simulink model "SimulacionPenduloSimpleFuzzyController"  (R2024b)
settings: Solver=ode45  StartTime=0.0  StopTime=20  RelTol=1e-3
libraries: fuzblock x1
settings Model: Creator=Lenovo  LastModifiedBy=Lenovo

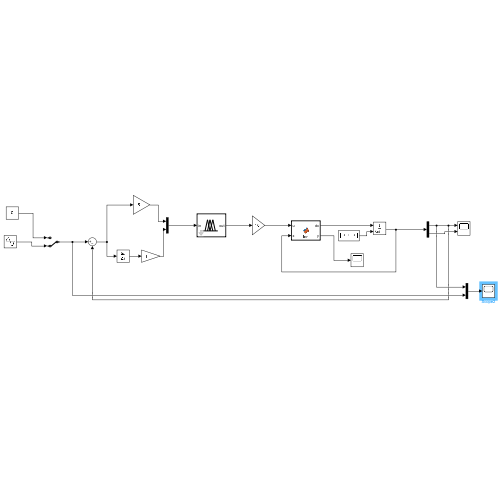
[thumbnail: Simulink's stored preview of the top-level diagram]
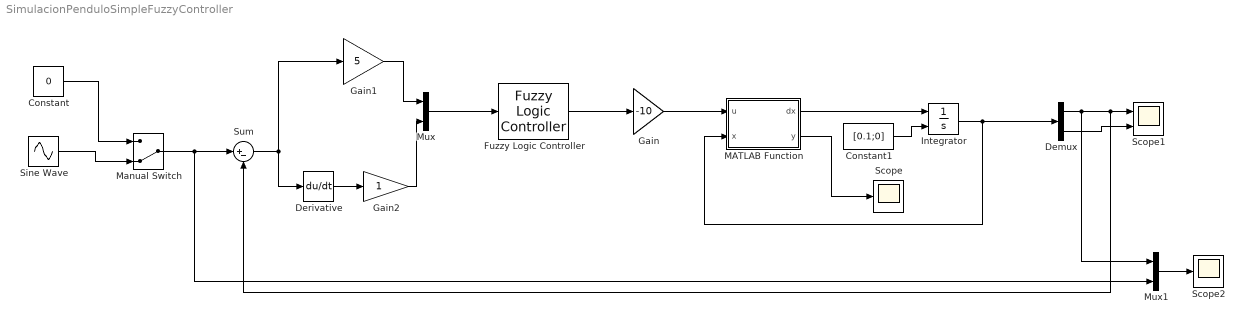
== system SimulacionPenduloSimpleFuzzyController ==
  Constant : Constant  Value=0
  Constant1 : Constant  Value=[0.1;0]
  Demux : Demux  Outputs=2
  Derivative : Derivative
  Fuzzy Logic Controller : fuzblock/Fuzzy Logic  Controller  FIS='D:\02. UP\Especialidad 1\Control difuso\Semana 05\Fuzzy5x5.fis'  OutputSampleNumber=101  DataType=double  FuzzifiedInputs=off  RuleFiringStrengths=off  RuleOutputs=off  AggregatedOutputs=off  SimulateUsing=Interpreted execution  OutOfRangeInputValueMessage=warning  NoRuleFiredMessage=warning  EmptyOutputFuzzySetMessage=warning
  Gain : Gain  Gain=-10
  Gain1 : Gain  Gain=5
  Gain2 : Gain
  Integrator : Integrator  InitialConditionSource=external
  MATLAB Function : MATLAB Function  TreatAsAtomicUnit=on
  Manual Switch : ManualSwitch  CurrentSetting=0
  Mux : Mux  Inputs=2
  Mux1 : Mux  Inputs=2
  Scope : Scope
  Scope1 : Scope  NumInputPorts=2
  Scope2 : Scope
  Sine Wave : Sin  Amplitude=.25  Frequency=4  SampleTime=0
  Sum : Sum  Inputs=|+-
  wires:
  Integrator/1 -> Demux/1, MATLAB Function/2(x)
  MATLAB Function/1(dx) -> Integrator/1
  Constant1/1 -> Integrator/2
  Demux/1 -> Mux1/1, Sum/2, Scope1/1
  Demux/2 -> Scope1/2
  MATLAB Function/2(y) -> Scope/1
  Gain/1 -> MATLAB Function/1(u)
  Fuzzy Logic Controller/1 -> Gain/1
  Mux/1 -> Fuzzy Logic Controller/1
  Gain1/1 -> Mux/1
  Gain2/1 -> Mux/2
  Derivative/1 -> Gain2/1
  Sum/1 -> Derivative/1, Gain1/1
  Manual Switch/1 -> Mux1/2, Sum/1
  Constant/1 -> Manual Switch/1
  Sine Wave/1 -> Manual Switch/2
  Mux1/1 -> Scope2/1

== matlab function SimulacionPenduloSimpleFuzzyController/MATLAB Function ==
  data: dx output; u input; y output; x input
function [dx, y] = fcn(u,x)

l=1; m=1; g=9.81; b=0.5; I=m*l^2;
x1=x(1);
x2=x(2);
dx1=x2;
dx2=-g/l*sin(x1)-(b*l/I)*x2+u/I;
dx = [dx1;dx2];

y = x1;
